simulink model "System_model_discrete"  (R2024b)
settings: Solver=FixedStepDiscrete  StartTime=0.0  StopTime=T_final  FixedStep=T_sample  RelTol=1e-3
values from neighbouring files (symbols this model uses):
  BDD_thresh = 0.5e-1    (= 0.05)    [run_model.m]
  C_obsv_d = C_obsv    [run_model.m]
  D_obsv_d = D_obsv    [run_model.m]
  l = n_input    [run_model.m]
  L_obsv = place(A_bar_d.',C_obsv_d.',P).'    [run_model.m]
  load_buses = ones(n_bus-n_gen,1)    [run_model.m]
  m = n_meas    [run_model.m]
  max_attack = 0    [run_model.m]
  n = n_states    [run_model.m]
  n_attack = round(0.3*n_input)    [run_model.m]
  n_gen = size(gen,1)    [run_model.m]
  n_load = n_bus-n_gen    [run_model.m]
  n_meas = n_gen + n_bus + 1    [run_model.m]
  n_states = 2*n_gen    [run_model.m]
  r_tau = max(sum(Sigma_inv_k*(error.^2)))    [run_model.m]
  Sigma_inv_k = diag(sigma_inv_k)    [run_model.m]
  sigma_inv_k = 1e4*(3 + 2*rand(m,1))    [run_model.m]
  T = round(2*n)    [run_model.m]
  T_sample = 0.01    [run_model.m]
  T_start_attack = .2*T_final    (= 1.6)    [run_model.m]
  T_start_opt = T_final*2    (= 16)    [run_model.m]
  U0 = zeros(l,T)    [run_model.m]
  U_y_1 = zeros(n_meas,n_comp)    [run_model.m]
  x0 = zeros(n_states,1)    [run_model.m]
  Y0 = zeros(m,T)    [run_model.m]
  z_0 = zeros(n+m*T,1)    [run_model.m]
undefined symbols (not defined in the file or in its folder): A_bar_d, B_bar_d, G_T, HT, PhiT, sigbuilder_block, Theta_T
libraries: simulink x4
settings Model: Creator=oanubi  LastModifiedBy=oanubi
settings SolverCC: AlgebraicLoopSolver=TrustRegion
settings DebuggingCC: UnconnectedInputMsg=warning  UnconnectedOutputMsg=warning  UnconnectedLineMsg=warning
settings ModelReferenceCC: EnableRefExpFcnMdlSchedulingChecks=on
settings RTWCC: GPUComputeCapability=3.5

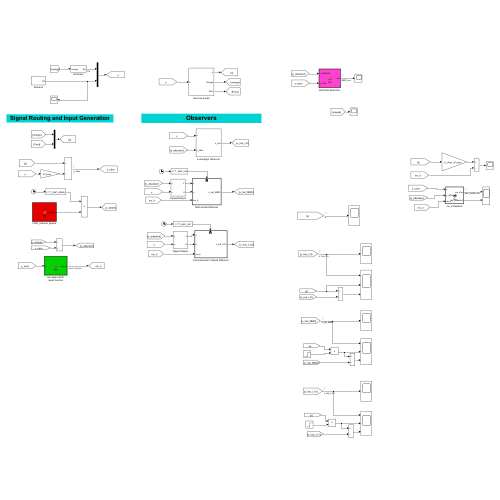
[thumbnail: Simulink's stored preview of the top-level diagram]
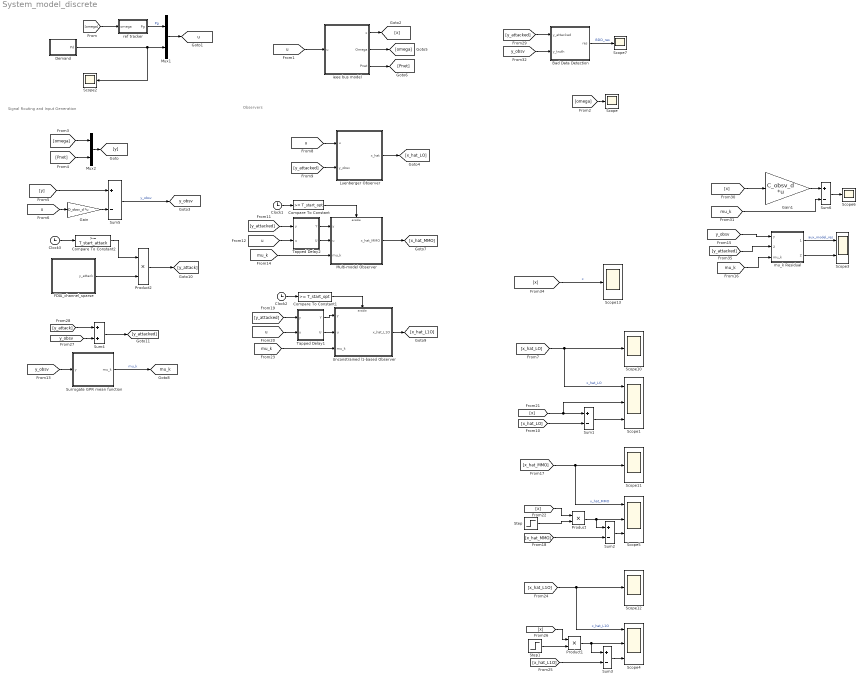
== system System_model_discrete ==
  note: Observers
  note: Signal Routing and Input Generation
  Bad Data Detection : MATLAB Function  TreatAsAtomicUnit=on
  Clock1 : Clock
  Clock2 : Clock
  Clock3 : Clock
  Compare To Constant : simulink/Logic and Bit Operations/Compare To Constant  relop=>=  const=T_start_opt  OutDataTypeStr=boolean
  Compare To Constant1 : simulink/Logic and Bit Operations/Compare To Constant  relop=>=  const=T_start_opt  OutDataTypeStr=boolean
  Compare To Constant2 : simulink/Logic and Bit Operations/Compare To Constant  relop=>=  const=T_start_attack  OutDataTypeStr=boolean
  Demand : Subsystem
  FDIA_channel_sparse : MATLAB Function  TreatAsAtomicUnit=on
  Gain : Gain  Gain=D_obsv_d  Multiplication=Matrix(K*u) (u vector)
  Gain1 : Gain  Gain=C_obsv_d  Multiplication=Matrix(K*u) (u vector)
  Luenberger Observer : Subsystem
  Multi-model Observer : Subsystem
  Mux1 : Mux  Inputs=2
  Mux2 : Mux  Inputs=2
  Product : Product
  Product1 : Product
  Product2 : Product
  Scope{,2,6..7,10..13} (8 alike) : Scope
  Scope1 : Scope  NumInputPorts=3
  Scope3 : Scope  NumInputPorts=2
  Scope4 : Scope  NumInputPorts=3
  Scope5 : Scope  NumInputPorts=3
  Step : Step  Time=1.5*T*T_sample  SampleTime=0
  Step1 : Step  Time=1.5*T*T_sample  SampleTime=0
  Sum{1..3,5..6} (5 alike) : Sum  Inputs=+-
  Sum4 : Sum
  Surrogate GPR mean function : MATLAB Function  TreatAsAtomicUnit=on
  Tapped Delay1 : Subsystem
  Tapped Delay2 : Subsystem
  Unconstrained l1-based Observer : Subsystem
  ieee bus model : Subsystem
  mu_k Residual : MATLAB Function  TreatAsAtomicUnit=on
  ref tracker : Subsystem
  tag scope: mu_k=global, u=global, y_obsv=global
  wires:
  [u] -> ieee bus model/1(u)
  Demand/1(Pd) -> Scope2/1, Mux1/2
  ref tracker/1(Pg) -> Mux1/1  "Pg"
  Mux1/1 -> [u]
  ieee bus model/2(Omega) -> [omega]
  ieee bus model/1(x) -> [x]
  ieee bus model/3(Pnet) -> [Pnet]
  [omega] -> ref tracker/1(omega)
  [omega] -> Scope/1
  Mux2/1 -> [y]
  [omega] -> Mux2/1
  [Pnet] -> Mux2/2
  [y] -> Sum5/1
  Gain/1 -> Sum5/2
  [u] -> Gain/1
  Sum5/1 -> [y_obsv]  "y_obsv"
  [u] -> Luenberger Observer/1(u)
  [y_attacked] -> Luenberger Observer/2(y_obsv)
  Luenberger Observer/1(x_hat) -> [x_hat_LO]
  Tapped Delay2/2(U) -> Multi-model Observer/2(u)
  Tapped Delay2/1(Y) -> Multi-model Observer/1(y)
  [u] -> Tapped Delay2/2(u)
  Clock1/1 -> Compare To Constant/1
  [y_attacked] -> Tapped Delay2/1(y)
  Compare To Constant/1 -> Multi-model Observer/Enable
  [y_obsv] -> Surrogate GPR mean function/1(y)
  Surrogate GPR mean function/1(mu_k) -> [mu_k]  "mu_k"
  [mu_k] -> Multi-model Observer/3(mu_k)
  [mu_k] -> mu_k Residual/3(mu_k)
  mu_k Residual/1(res_true) -> Scope3/1  "aux_model_res"
  [x_hat_MMO] -> Sum2/2
  [x_hat_LO] -> Sum1/2
  [x] -> Sum1/1, Scope1/2
  Sum1/1 -> Scope1/3
  Sum2/1 -> Scope5/3
  Multi-model Observer/1(x_hat_MMO) -> [x_hat_MMO]
  Unconstrained l1-based Observer/1(x_hat_L1O) -> [x_hat_L1O]
  [y_attacked] -> Tapped Delay1/1(y)
  Tapped Delay1/1(Y) -> Unconstrained l1-based Observer/1(y)
  [u] -> Tapped Delay1/2(u)
  Clock2/1 -> Compare To Constant1/1
  Tapped Delay1/2(U) -> Unconstrained l1-based Observer/2(u)
  Compare To Constant1/1 -> Unconstrained l1-based Observer/Enable
  [mu_k] -> Unconstrained l1-based Observer/3(mu_k)
  Sum3/1 -> Scope4/3
  [x_hat_L1O] -> Sum3/2
  [y_obsv] -> Sum4/2
  Sum4/1 -> [y_attacked]
  [y_attack] -> Sum4/1
  [x] -> Product/1
  Step/1 -> Product/2
  Product/1 -> Sum2/1, Scope5/2
  [x] -> Product1/1
  Step1/1 -> Product1/2
  Product1/1 -> Sum3/1, Scope4/2
  Gain1/1 -> Sum6/1
  [x] -> Gain1/1
  [mu_k] -> Sum6/2
  Sum6/1 -> Scope6/1
  [y_obsv] -> mu_k Residual/1(y)
  [y_attacked] -> Bad Data Detection/1(y_attacked)
  Bad Data Detection/1(res) -> Scope7/1  "BDD_res"
  [y_obsv] -> Bad Data Detection/2(y_truth)
  [x_hat_LO] -> Scope10/1, Scope1/1  "x_hat_LO"
  [x_hat_MMO] -> Scope5/1, Scope11/1  "x_hat_MMO"
  [x_hat_L1O] -> Scope4/1, Scope12/1  "x_hat_L1O"
  Product2/1 -> [y_attack]
  Compare To Constant2/1 -> Product2/1
  Clock3/1 -> Compare To Constant2/1
  mu_k Residual/2(res_attacked) -> Scope3/2
  [y_attacked] -> mu_k Residual/2(y_attacked)
  [x] -> Scope13/1  "x"
  FDIA_channel_sparse/1(y_attack) -> Product2/2

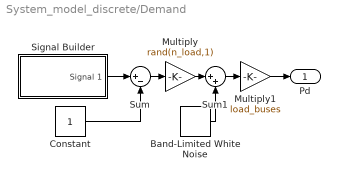
== system System_model_discrete/Demand ==
  Band-Limited White Noise : simulink/Sources/Band-Limited White Noise  Cov=1e-8  Ts=0.1  seed=[23341]
  Constant : Constant
  Multiply : Gain  Gain=rand(n_load,1)
  Multiply1 : Gain  Gain=load_buses
  Signal Builder : Subsystem  Tag=STV Subsys  LoadFcn=sigbuilder_block('load');  StartFcn=sigbuilder_block('start');  StopFcn=sigbuilder_block('stop');  ClipboardFcn=sigbuilder_block('clipboard');  mask(Sigbuilder block){tuvar=[0:10]}
      mask help: Simulink:masks:SigbuilderBlock_MD
      mask init:
      | if ~strcmp(get_param(bdroot(gcbh),'SimulationStatus'),'stopped') tuvar = sigbuilder_block('maskInit'); end
      settings: CopyFcn=sigbuilder_block('copy');  DeleteFcn=sigbuilder_block('delete');  ModelCloseFcn=sigbuilder_block('modelClose');  PreSaveFcn=sigbuilder_block('preSave');  PauseFcn=sigbuilder_block('pause');  ContinueFcn=sigbuilder_block('continue');  NameChangeFcn=sigbuilder_block('namechange');  OpenFcn=sigbuilder_block('open',[439.2 145.2 550.2 399.9 ]);  CloseFcn=sigbuilder_block('close');
      mask Display: plot(0, 0, 100, 100,[2, 2, 32, 32, 2], [68, 8, 8, 68, 68],[32, 2], [38, 38], [32, 19, 2],[53, 60, 44], [32, 17, 17, 2],[16, 16, 31, 31]);txt = getActiveGroup(gcbh);text(2, 100, txt,'verticalAlignment', 'top');
  Sum : Sum  Inputs=|+-
  Sum1 : Sum  Inputs=|++
  Pd : Outport
  wires:
  Sum/1 -> Multiply/1
  Signal Builder/1(Signal 1) -> Sum/1
  Constant/1 -> Sum/2
  Multiply/1 -> Sum1/1
  Band-Limited White Noise/1 -> Sum1/2
  Sum1/1 -> Multiply1/1
  Multiply1/1 -> Pd/1

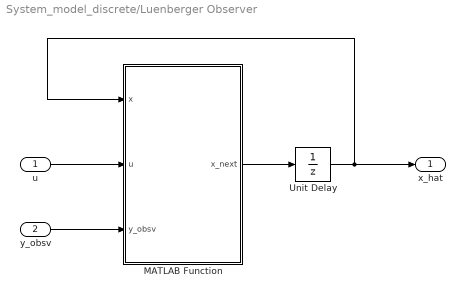
== system System_model_discrete/Luenberger Observer ==
  u : Inport
  y_obsv : Inport  Port=2
  MATLAB Function : MATLAB Function  TreatAsAtomicUnit=on
  Unit Delay : UnitDelay  InitialCondition=zeros(n_states,1)  SampleTime=-1  HasFrameUpgradeWarning=on
  x_hat : Outport
  wires:
  MATLAB Function/1(x_next) -> Unit Delay/1
  Unit Delay/1 -> x_hat/1, MATLAB Function/1(x)
  u/1 -> MATLAB Function/2(u)
  y_obsv/1 -> MATLAB Function/3(y_obsv)

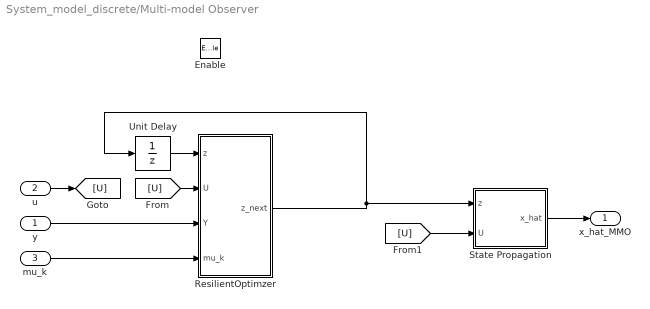
== system System_model_discrete/Multi-model Observer ==
  y : Inport
  u : Inport  Port=2
  mu_k : Inport  Port=3
  Enable : EnablePort
  ResilientOptimzer : MATLAB Function  TreatAsAtomicUnit=on
  State Propagation : MATLAB Function  TreatAsAtomicUnit=on
  Unit Delay : UnitDelay  InitialCondition=z_0  SampleTime=-1  HasFrameUpgradeWarning=on
  x_hat_MMO : Outport
  wires:
  mu_k/1 -> ResilientOptimzer/4(mu_k)
  ResilientOptimzer/1(z_next) -> State Propagation/1(z), Unit Delay/1
  u/1 -> [U]
  y/1 -> ResilientOptimzer/3(Y)
  [U] -> ResilientOptimzer/2(U)
  [U] -> State Propagation/2(U)
  State Propagation/1(x_hat) -> x_hat_MMO/1
  Unit Delay/1 -> ResilientOptimzer/1(z)

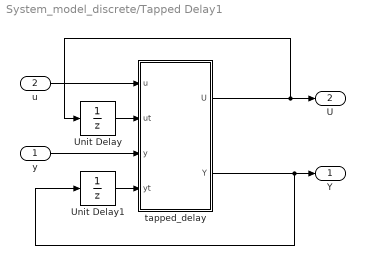
== system System_model_discrete/Tapped Delay1 ==
  y : Inport
  u : Inport  Port=2
  Unit Delay : UnitDelay  InitialCondition=U0  SampleTime=-1  HasFrameUpgradeWarning=on
  Unit Delay1 : UnitDelay  InitialCondition=Y0  SampleTime=-1  HasFrameUpgradeWarning=on
  tapped_delay : MATLAB Function  TreatAsAtomicUnit=on
  Y : Outport
  U : Outport  Port=2
  wires:
  u/1 -> tapped_delay/1(u)
  y/1 -> tapped_delay/3(y)
  tapped_delay/1(U) -> Unit Delay/1, U/1
  tapped_delay/2(Y) -> Unit Delay1/1, Y/1
  Unit Delay/1 -> tapped_delay/2(ut)
  Unit Delay1/1 -> tapped_delay/4(yt)

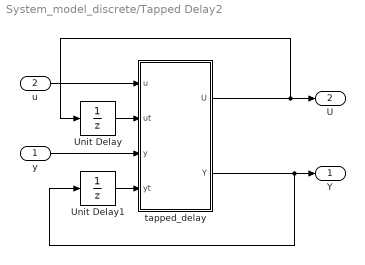
== system System_model_discrete/Tapped Delay2 ==
  y : Inport
  u : Inport  Port=2
  Unit Delay : UnitDelay  InitialCondition=U0  SampleTime=-1  HasFrameUpgradeWarning=on
  Unit Delay1 : UnitDelay  InitialCondition=Y0  SampleTime=-1  HasFrameUpgradeWarning=on
  tapped_delay : MATLAB Function  TreatAsAtomicUnit=on
  Y : Outport
  U : Outport  Port=2
  wires:
  tapped_delay/2(Y) -> Y/1, Unit Delay1/1
  tapped_delay/1(U) -> U/1, Unit Delay/1
  y/1 -> tapped_delay/3(y)
  u/1 -> tapped_delay/1(u)
  Unit Delay/1 -> tapped_delay/2(ut)
  Unit Delay1/1 -> tapped_delay/4(yt)

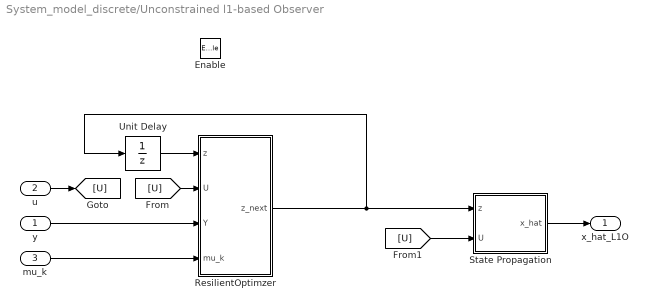
== system System_model_discrete/Unconstrained l1-based Observer ==
  y : Inport
  u : Inport  Port=2
  mu_k : Inport  Port=3
  Enable : EnablePort
  ResilientOptimzer : MATLAB Function  TreatAsAtomicUnit=on
  State Propagation : MATLAB Function  TreatAsAtomicUnit=on
  Unit Delay : UnitDelay  InitialCondition=z_0  SampleTime=-1  HasFrameUpgradeWarning=on
  x_hat_L1O : Outport
  wires:
  mu_k/1 -> ResilientOptimzer/4(mu_k)
  ResilientOptimzer/1(z_next) -> State Propagation/1(z), Unit Delay/1
  u/1 -> [U]
  y/1 -> ResilientOptimzer/3(Y)
  [U] -> ResilientOptimzer/2(U)
  [U] -> State Propagation/2(U)
  State Propagation/1(x_hat) -> x_hat_L1O/1
  Unit Delay/1 -> ResilientOptimzer/1(z)

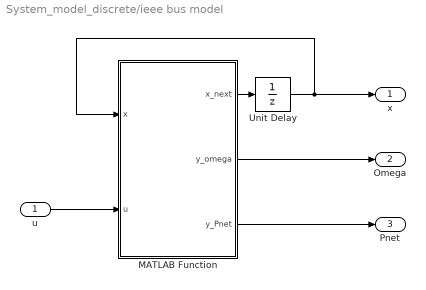
== system System_model_discrete/ieee bus model ==
  u : Inport
  MATLAB Function : MATLAB Function  TreatAsAtomicUnit=on
  Unit Delay : UnitDelay  InitialCondition=x0  SampleTime=-1  HasFrameUpgradeWarning=on
  x : Outport
  Omega : Outport  Port=2
  Pnet : Outport  Port=3
  wires:
  MATLAB Function/1(x_next) -> Unit Delay/1
  Unit Delay/1 -> x/1, MATLAB Function/1(x)
  u/1 -> MATLAB Function/2(u)
  MATLAB Function/2(y_omega) -> Omega/1
  MATLAB Function/3(y_Pnet) -> Pnet/1

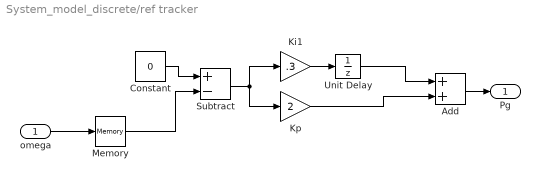
== system System_model_discrete/ref tracker ==
  omega : Inport
  Add : Sum
  Constant : Constant  Value=0
  Ki1 : Gain  Gain=.3
  Kp : Gain  Gain=2
  Memory : Memory  InitialCondition=zeros(n_gen,1)
  Subtract : Sum  Inputs=+-
  Unit Delay : UnitDelay  InitialCondition=zeros(n_gen,1)  SampleTime=-1  HasFrameUpgradeWarning=on
  Pg : Outport
  wires:
  Kp/1 -> Add/2
  Unit Delay/1 -> Add/1
  Add/1 -> Pg/1
  Constant/1 -> Subtract/1
  Subtract/1 -> Ki1/1, Kp/1
  Ki1/1 -> Unit Delay/1
  Memory/1 -> Subtract/2
  omega/1 -> Memory/1

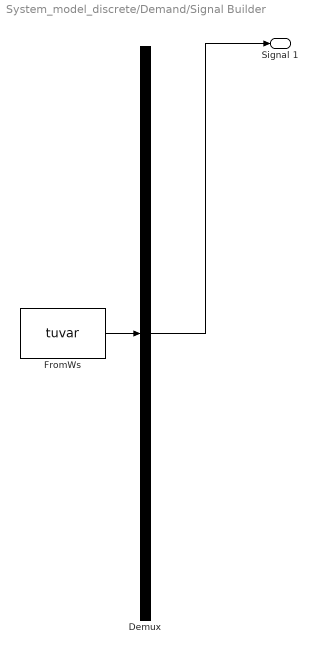
== system System_model_discrete/Demand/Signal Builder ==
  Demux : Demux  Tag=STV Demux  Outputs=1
      settings: DisplayOption=none
  FromWs : FromWorkspace  Tag=STV FromWs  VariableName=tuvar
      SigBuilderData=|
      | common.afterFinalStr = 'Extrapolate'
      | common.sampleTime = 0
      | dataSet.timeRange = [0 10]
      | dataSet.name = 'Group 1'
      | sbobj.Groups.Name = 'Group 1'
      | sbobj.Groups.Signals.Name = 'Signal 1'
      | sbobj.Groups.Signals.XData = [0 0.46 1.5 2.5 4 5 6 7 10]
      | sbobj.Groups.Signals.YData = [1 1.106 1.2 1.2 0.8 0.8 1 1 1]
  Signal 1 : Outport  Tag=STV Outport
  wires:
  Demux/1 -> Signal 1/1
  FromWs/1 -> Demux/1

== matlab function System_model_discrete/Multi-model Observer/State Propagation ==
  data: z input; x_hat output; U input; Theta_T parameter; G_T parameter; n parameter; T parameter; l parameter
function x_hat = fcn(z,U,Theta_T, G_T,n,T,l)
% x_hat = fcn(z,U,PhiT, HT,n_states)
% Propagates the estimated intial state to the current time
u_local = zeros(l,T-1);
u_local(:,:) = U(:,1:end-1);


% State propagation
x_hat = Theta_T*z(1:n) + G_T*u_local(:);

== matlab function System_model_discrete/Unconstrained l1-based Observer/ResilientOptimzer ==
  data: z input; z_next output; U input; Y input; mu_k input; Sigma_inv_k parameter; HT parameter; PhiT parameter; r_tau parameter; n_states parameter; l parameter; T parameter; n_meas parameter
function z_next  = fcn(z,U,Y,mu_k,Sigma_inv_k, HT, PhiT, r_tau, n_states,l,T,n_meas)
u_local = zeros(l,T-1);
u_local(:,:) = U(:,1:end-1);
% vectorized
u = u_local(:);
y = Y(:);

coder.extrinsic('solver_call_unc')
z_next = zeros(n_states + n_meas*T,1);
z_next(:) = solver_call_unc(y,u,mu_k,Sigma_inv_k,z,HT,PhiT,r_tau);

== matlab function System_model_discrete/Unconstrained l1-based Observer/State Propagation ==
  data: z input; x_hat output; U input; Theta_T parameter; G_T parameter; n parameter; T parameter; l parameter
function x_hat = fcn(z,U,Theta_T, G_T,n,T,l)
% x_hat = fcn(z,U,PhiT, HT,n_states)
% Propagates the estimated intial state to the current time
u_local = zeros(l,T-1);
u_local(:,:) = U(:,1:end-1);


% State propagation
x_hat = Theta_T*z(1:n) + G_T*u_local(:);

== matlab function System_model_discrete/Tapped Delay1/tapped_delay ==
  data: u input; U output; ut input; y input; yt input; Y output
function [U,Y] = fcn(u,ut,y,yt)
%% tapped_delay_array
% shift columns from tapped matrix to the left and appends most recent
% vector to the last column
%%% input
ut(:,1:end-1) = ut(:,2:end);
ut(:,end) = u;
U = ut;
%%% output
yt(:,1:end-1) = yt(:,2:end);
yt(:,end) = y;
Y = yt;

== matlab function System_model_discrete/FDIA_channel_sparse ==
  data: n_attack parameter; y_attack output; n_meas parameter; C_obsv_d parameter; max_attack parameter; BDD_thresh parameter
function y_attack = fcn(n_attack,n_meas,C_obsv_d,max_attack, BDD_thresh)

%% Measurement Channel Attack
%  Assumptions:
%  1. The attacker knows the actual measurement
%  2. The attacker can only corrupt upto n_attack measurements
%  3. The attacker knows the BDD theshold

attack_idx = randi(n_meas,n_attack,1);
y_attack   = gen_attack_channel(C_obsv_d, max_attack,attack_idx,0.75*BDD_thresh);
                                                        % NOTE THE .75
                                                        % Used
                                                        % conservatively

== matlab function System_model_discrete/Bad Data Detection ==
  data: y_attacked input; y_truth input; res output; U2 parameter
function res = fcn(y_attacked,y_truth,U2)

res = [norm(U2.'*y_attacked,2);
       norm(U2.'*y_truth,2)];

== matlab function System_model_discrete/Luenberger Observer/MATLAB Function ==
  data: x input; x_next output; u input; y_obsv input; L_obsv parameter; A_bar_d parameter; C_obsv_d parameter; B_bar_d parameter
function x_next  = fcn(x,u,y_obsv,L_obsv,A_bar_d,C_obsv_d,B_bar_d)
% Discrete state-space model for system

x_next = A_bar_d*x + B_bar_d*u + L_obsv*(y_obsv - C_obsv_d*x);

== matlab function System_model_discrete/ieee bus model/MATLAB Function ==
  data: x input; x_next output; u input; y_omega output; A_bar_d parameter; C_obsv_d parameter; B_bar_d parameter; D_obsv_d parameter; n_gen parameter; n_meas parameter; y_Pnet output
function [x_next,y_omega,y_Pnet] = fcn(x,u,A_bar_d,C_obsv_d,B_bar_d,D_obsv_d,n_gen,n_meas)
% Discrete state-space model for system

x_next = A_bar_d*x + B_bar_d*u;

y = C_obsv_d*x + D_obsv_d*u;

y_omega = y(1:n_gen);
y_Pnet = y(n_gen+1:n_meas);

== matlab function System_model_discrete/Multi-model Observer/ResilientOptimzer ==
  data: z input; z_next output; U input; Y input; mu_k input; Sigma_inv_k parameter; HT parameter; PhiT parameter; r_tau parameter; n_states parameter; l parameter; T parameter; n_meas parameter
function z_next  = fcn(z,U,Y,mu_k,Sigma_inv_k, HT, PhiT, r_tau, n_states,l,T,n_meas)
u_local = zeros(l,T-1);
u_local(:,:) = U(:,1:end-1);
% vectorized
u = u_local(:);
y = Y(:);

coder.extrinsic('solver_call')
z_next = zeros(n_states + n_meas*T,1);
z_next(:) = solver_call(y,u,mu_k,Sigma_inv_k,z,HT,PhiT,r_tau);

== matlab function System_model_discrete/mu_k Residual ==
  data: y input; y_attacked input; res_true output; mu_k input; Sigma_inv_k parameter; r_tau parameter; res_attacked output
function [res_true,res_attacked] = fcn(y,y_attacked,mu_k,Sigma_inv_k, r_tau)

res_true = r_tau - (y-mu_k).'*Sigma_inv_k*(y-mu_k);
res_attacked = r_tau - (y_attacked-mu_k).'*Sigma_inv_k*(y_attacked-mu_k);

== matlab function System_model_discrete/Surrogate GPR mean function ==
  data: y input; mu_k output; sigma_inv_k parameter; r_tau parameter; m parameter; U_y_1 parameter
function mu_k = fcn(y,sigma_inv_k, r_tau,m,U_y_1)
% Prunes a random vector to find mu_k so that ||y-mu_k||_Sigma_inv_k <= r_tau

% first: random vector, secomd: normalize
y_rand = rand(m,1);
y_rand = sqrt(r_tau/max(sigma_inv_k))/norm(y_rand)*y_rand;

% create mu_k from y
mu_k = y - y_rand;

% mu_k = (U_y_1*U_y_1.')*y;

== matlab function System_model_discrete/Tapped Delay2/tapped_delay ==
  data: u input; U output; ut input; y input; yt input; Y output
function [U,Y] = fcn(u,ut,y,yt)
%% tapped_delay_array
% shift columns from tapped matrix to the left and appends most recent
% vector to the last column
%%% input
ut(:,1:end-1) = ut(:,2:end);
ut(:,end) = u;
U = ut;
%%% output
yt(:,1:end-1) = yt(:,2:end);
yt(:,end) = y;
Y = yt;
